simulink model "platform"  (R2023b)
settings: Solver=FixedStepAuto  StartTime=0.0  StopTime=time_end  FixedStep=0.001  RelTol=1e-3  EnableMultiTasking=on
values from neighbouring files (symbols this model uses):
  A = -2/((d1-d2)^3)    [collisioncon.m]    (also in main.m = [zeros(2 * M, 2 * M) eye(2 * M); zeros(2 * M, 2 * M) l * eye; mytunnel.m)
  B = 3*(d1+d2)/((d1-d2)^3)    [collisioncon.m]    (also in main.m = [zeros(2 * M, 2 * M); -l * eye(2 * M)]; mytunnel.m)
  C = -6*d1*d2/((d1-d2)^3)    [collisioncon.m]    (also in main.m = eye(4 * M); mytunnel.m)
  D = d2^2*(3*d1-d2)/((d1-d2)^3)    [collisioncon.m]    (also in main.m = zeros(4 * M, 2 * M); mytunnel.m)
  Initialcondition = [InitialPosition; zeros(2 * M, 1)]    [main.m]
  InitialPosition = [InitialPosition;UavTeam.Uav(k).CurrentPos]    [UAVInitialization.m]
  M = UavTeam.AvailableNumMax    [MyMap.m]    (also in collisioncon.m; dangerdistance.m; main.m = 40)
  UavTeam = UAVInitialization(M, rm)    [main.m]
settings Model: SimulationMode=accelerator  Creator=Furao  LastModifiedBy=GZY
settings SolverCC: AlgebraicLoopSolver=TrustRegion
settings DataIOCC: LimitDataPoints=on  SaveFormat=Array  ReturnWorkspaceOutputs=off  SignalLoggingName=sigsOut
settings DebuggingCC: SaveWithParameterizedLinksMsg=none  UnderspecifiedInitializationDetection=Classic  MergeDetectMultiDrivingBlocksExec=none  SignalResolutionControl=TryResolveAllWithWarning  MultiTaskDSMMsg=warning  MultiTaskCondExecSysMsg=none  UnconnectedInputMsg=warning  UnconnectedOutputMsg=warning  UnconnectedLineMsg=warning  ArithmeticOperatorsInVariantConditions=warning
settings HardwareCC: ProdBitPerPointer=32  ProdBitPerSizeT=32  ProdBitPerPtrDiffT=32  ProdLargestAtomicFloat=None  ProdIntDivRoundTo=Undefined  ProdEndianess=Unspecified  ProdWordSize=32  ProdHWDeviceType=32-bit Generic  TargetUnknown=on
settings ModelReferenceCC: EnableRefExpFcnMdlSchedulingChecks=on  PropagateSignalLabelsOutOfModel=off
settings SFSimCC: SimUseLocalCustomCode=off  CustomCodeUndefinedFunction=UseInterfaceOnly
settings RTWCC: RTWUseLocalCustomCode=off
settings CodeAppCC: StateflowObjectComments=on
settings GRTTargetCC: TargetLangStandard=C89/C90 (ANSI)  CombineOutputUpdateFcns=off  GRTInterface=on
settings ConfigComp: CovMetricSettings=dw  CovSaveCumulativeToWorkspaceVar=on  CovSaveSingleToWorkspaceVar=on  CovExternalEMLEnable=off

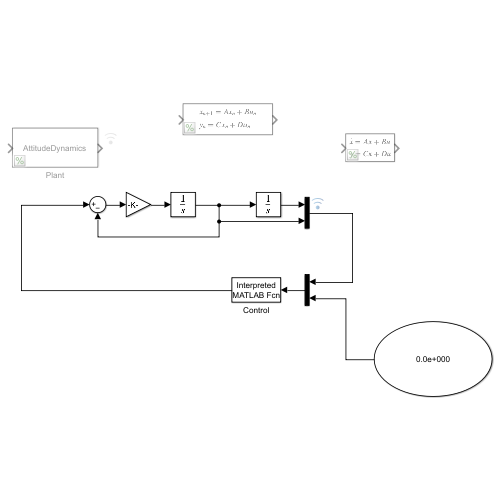
[thumbnail: Simulink's stored preview of the top-level diagram]
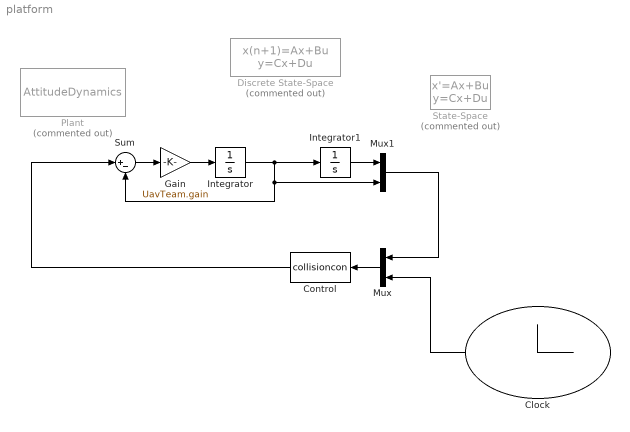
== system platform ==
  Clock : Clock
  Control : MATLABFcn  MATLABFcn=collisioncon
  Discrete State-Space : DiscreteStateSpace  Commented=on  A=A  B=B  C=C  D=D  InitialCondition=Initialcondition  SampleTime=-1
  Gain : Gain  Gain=UavTeam.gain
  Integrator : Integrator  InitialCondition=zeros(2*M,1)
  Integrator1 : Integrator  InitialCondition=InitialPosition
  Mux : Mux  Inputs=2
  Mux1 : Mux  Inputs=2
  Plant : S-Function  Commented=on  FunctionName=AttitudeDynamics  SFunctionDeploymentMode=off  EnableBusSupport=off
  State-Space : StateSpace  Commented=on  A=A  B=B  C=C  D=D  InitialCondition=Initialcondition
  Sum : Sum  Inputs=|+-
  wires:
  Mux/1 -> Control/1
  Clock/1 -> Mux/2
  Control/1 -> Sum/1
  Sum/1 -> Gain/1
  Gain/1 -> Integrator/1
  Mux1/1 -> Mux/1
  Integrator1/1 -> Mux1/1
  Integrator/1 -> Mux1/2, Sum/2, Integrator1/1
